simulink model "Exercise_4"  (R2022a)
settings: Solver=VariableStepAuto  StartTime=0.0  StopTime=10.0  RelTol=1e-3
libraries: simulink x1
settings Model: Creator=Shocky  LastModifiedBy=Shocky

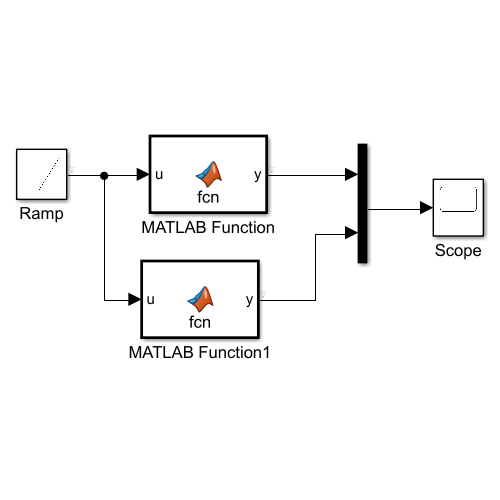
[thumbnail: Simulink's stored preview of the top-level diagram]
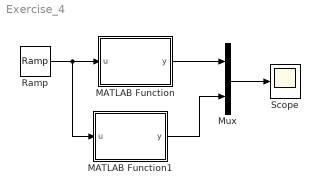
== system Exercise_4 ==
  MATLAB Function : MATLAB Function  TreatAsAtomicUnit=on
  MATLAB Function1 : MATLAB Function  TreatAsAtomicUnit=on
  Mux : Mux  Inputs=2
  Ramp : simulink/Sources/Ramp  slope=1  start=0  InitialOutput=0
  Scope : Scope
  wires:
  MATLAB Function/1(y) -> Mux/1
  Mux/1 -> Scope/1
  MATLAB Function1/1(y) -> Mux/2
  Ramp/1 -> MATLAB Function/1(u), MATLAB Function1/1(u)

== matlab function Exercise_4/MATLAB Function ==
  data: u input; y output
function y = fcn(u)
y=sin(u);
end

== matlab function Exercise_4/MATLAB Function1 ==
  data: u input; y output
function y = fcn(u)
y=cos(u);
end
